simulink model "SecRwRtStFtrstTrgtPosSelc"  (R2018b)
settings: Solver=FixedStepDiscrete  StartTime=0.0  StopTime=10.0  FixedStep=0.01  RelTol=1e-3
undefined symbols (not defined in the file or in its folder): KeSMSw4SAcsMd24SecRwRtStFtrstUpwdDnwdPos_Val, KeSMSw4SAcsMd24SecRwRtStFtrstUpwdDnwdPosMax_Val, KeSMSw4SAcsMd24SecRwRtStFtrstUpwdDnwdPosMin_Val, KeSMSw4SAcsMd26SecRwRtStFtrstUpwdDnwdPos_Val, KeSMSw4SAcsMd26SecRwRtStFtrstUpwdDnwdPosMax_Val, KeSMSw4SAcsMd26SecRwRtStFtrstUpwdDnwdPosMin_Val, KeSMSw4SLegrstCloseMdSecRwRtStFtrstUpwdDnwdPos_Val, KeSMSw4SLegrstCloseMdSecRwRtStFtrstUpwdDnwdPosMax_Val, KeSMSw4SLegrstCloseMdSecRwRtStFtrstUpwdDnwdPosMin_Val, KeSMSw4SLegrstOpenMdSecRwRtStFtrstUpwdDnwdPos_Val, KeSMSw4SLegrstOpenMdSecRwRtStFtrstUpwdDnwdPosMax_Val, KeSMSw4SLegrstOpenMdSecRwRtStFtrstUpwdDnwdPosMin_Val, KeSMSw4sLyingMDSecRwRtStFtrstUpwdDnwdPos_Val, KeSMSw4sLyingMDSecRwRtStFtrstUpwdDnwdPosMax_Val, KeSMSw4sLyingMDSecRwRtStFtrstUpwdDnwdPosMin_Val, KeSMSw4sRecoveryMDSecRwRtStFtrstUpwdDnwdPos_Val, KeSMSw4sRecoveryMDSecRwRtStFtrstUpwdDnwdPosMax_Val, KeSMSw4sRecoveryMDSecRwRtStFtrstUpwdDnwdPosMin_Val, KeSMSw4sVIPMDSecRwRtStFtrstUpwdDnwdPos_Val, KeSMSw4sVIPMDSecRwRtStFtrstUpwdDnwdPosMax_Val, KeSMSw4sVIPMDSecRwRtStFtrstUpwdDnwdPosMin_Val
libraries: TrgtPosSelcLib x8
settings Model: ModifiedHistory=2023.8.1 V2.0.0 CR401790 增加模式21-26  Creator=sn2xws  LastModifiedBy=sn2xws
settings DataIOCC: SaveFormat=StructureWithTime
settings OptimizationCC: DefaultParameterBehavior=Inlined  EnhancedBackFolding=on  PassReuseOutputArgsAs=Individual arguments  ZeroExternalMemoryAtStartup=off  ZeroInternalMemoryAtStartup=off  OptimizeBlockOrder=speed  DifferentSizesBufferReuse=on  OptimizationCustomize=off
settings DebuggingCC: ParameterTunabilityLossMsg=error
settings ModelReferenceCC: ModelReferenceNumInstancesAllowed=Single
settings SFSimCC: MATLABDynamicMemAlloc=off
settings RTWCC: SystemTargetFile=autosar.tlc  GenCodeOnly=on  TemplateMakefile=ert_default_tmf  Description=AUTOSAR  GenerateReport=on  IncludeHyperlinkInReport=on  LaunchReport=on  GenerateTraceInfo=on  GenerateTraceReport=on  GenerateTraceReportSl=on  GenerateTraceReportSf=on  GenerateTraceReportEml=on
settings CodeAppCC: ForceParamTrailComments=on  IgnoreCustomStorageClasses=off  OperatorAnnotations=on  SimulinkDataObjDesc=on  SFDataObjDesc=on  InsertBlockDesc=on
settings STFCustomTargetCC: TargetLangStandard=C99 (ISO)  MultiwordLength=256  ParMdlRefBuildCompliant=on  CompOptLevelCompliant=on  IncludeMdlTerminateFcn=off  CombineOutputUpdateFcns=on  SuppressErrorStatus=on  ERTCustomFileBanners=on  SupportNonFinite=off  SupportComplex=off  SupportContinuousTime=off  SupportNonInlinedSFcns=off  RemoveResetFunc=on  MATLABClassNameForMDSCustomization=Simulink.SoftwareTarget.ERTCustomization  AutosarCompliant=on  UseToolchainInfoCompliant=on  LookupTableObjectStructAxisOrder=2,1,3,4,...  LUTObjectStructOrderEvenSpacing=Size,Table,Breakpoints  SystemTargetFile=autosar.tlc
settings ERTTargetCC: TargetLangStandard=C99 (ISO)  ConcurrentExecutionCompliant=off  IncludeMdlTerminateFcn=off  SuppressErrorStatus=on  SupportNonFinite=off  SupportComplex=off  ModelStepFunctionPrototypeControlCompliant=off  CPPClassGenCompliant=off  AutosarCompliant=on  LookupTableObjectStructAxisOrder=2,1,3,4,...  LUTObjectStructOrderEvenSpacing=Size,Table,Breakpoints  InlinedParameterPlacement=NonHierarchical  ERTCustomFileTemplate=example_file_process.tlc  ERTFilePackagingFormat=Compact

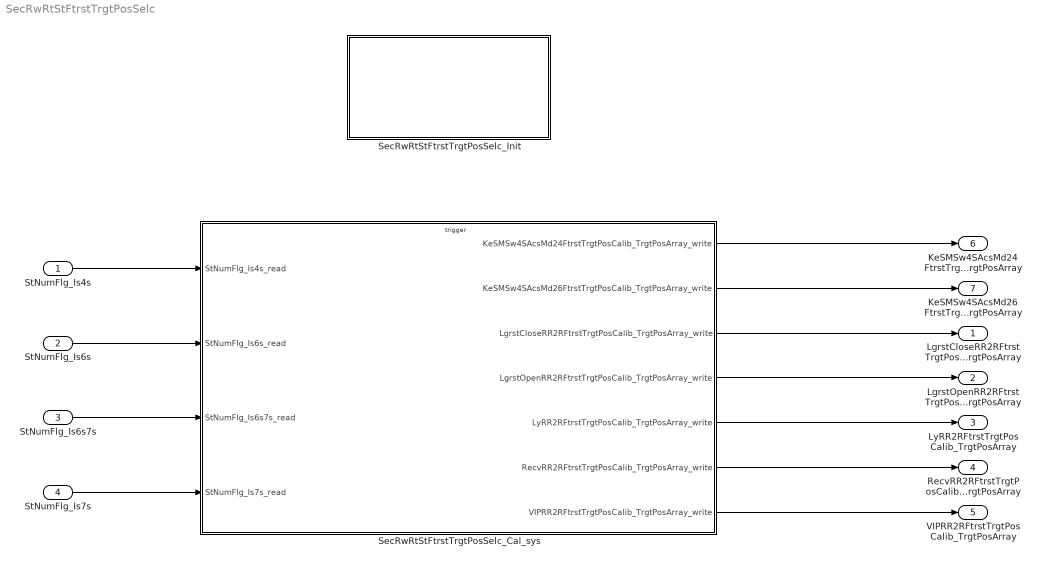
== system SecRwRtStFtrstTrgtPosSelc ==
  StNumFlg_Is4s : Inport  OutDataTypeStr=boolean  PortDimensions=1
  StNumFlg_Is6s : Inport  Port=2  OutDataTypeStr=boolean  PortDimensions=1
  StNumFlg_Is6s7s : Inport  Port=3  OutDataTypeStr=boolean  PortDimensions=1
  StNumFlg_Is7s : Inport  Port=4  OutDataTypeStr=boolean  PortDimensions=1
  SecRwRtStFtrstTrgtPosSelc_Cal_sys : Subsystem
  SecRwRtStFtrstTrgtPosSelc_Init : Subsystem
  LgrstCloseRR2RFtrstTrgtPosCalib_TrgtPosArray : Outport  Description=|  OutDataTypeStr=uint16  PortDimensions=3
      | 0:Pos
      | 1:Max
      | 2:Min
  LgrstOpenRR2RFtrstTrgtPosCalib_TrgtPosArray : Outport  Description=|  Port=2  OutDataTypeStr=uint16  PortDimensions=3
      | 0:Pos
      | 1:Max
      | 2:Min
  LyRR2RFtrstTrgtPosCalib_TrgtPosArray : Outport  Description=|  Port=3  OutDataTypeStr=uint16  PortDimensions=3
      | 0:Pos
      | 1:Max
      | 2:Min
  RecvRR2RFtrstTrgtPosCalib_TrgtPosArray : Outport  Description=|  Port=4  OutDataTypeStr=uint16  PortDimensions=3
      | 0:Pos
      | 1:Max
      | 2:Min
  VIPRR2RFtrstTrgtPosCalib_TrgtPosArray : Outport  Description=|  Port=5  OutDataTypeStr=uint16  PortDimensions=3
      | 0:Pos
      | 1:Max
      | 2:Min
  KeSMSw4SAcsMd24FtrstTrgtPosCalib_TrgtPosArray : Outport  Description=|  Port=6  OutDataTypeStr=uint16  PortDimensions=3
      | 0:Pos
      | 1:Max
      | 2:Min
  KeSMSw4SAcsMd26FtrstTrgtPosCalib_TrgtPosArray : Outport  Description=|  Port=7  OutDataTypeStr=uint16  PortDimensions=3
      | 0:Pos
      | 1:Max
      | 2:Min
  wires:
  StNumFlg_Is4s/1 -> SecRwRtStFtrstTrgtPosSelc_Cal_sys/1(StNumFlg_Is4s_read)
  StNumFlg_Is6s/1 -> SecRwRtStFtrstTrgtPosSelc_Cal_sys/2(StNumFlg_Is6s_read)
  StNumFlg_Is6s7s/1 -> SecRwRtStFtrstTrgtPosSelc_Cal_sys/3(StNumFlg_Is6s7s_read)
  StNumFlg_Is7s/1 -> SecRwRtStFtrstTrgtPosSelc_Cal_sys/4(StNumFlg_Is7s_read)
  SecRwRtStFtrstTrgtPosSelc_Cal_sys/3(LgrstCloseRR2RFtrstTrgtPosCalib_TrgtPosArray_write) -> LgrstCloseRR2RFtrstTrgtPosCalib_TrgtPosArray/1
  SecRwRtStFtrstTrgtPosSelc_Cal_sys/4(LgrstOpenRR2RFtrstTrgtPosCalib_TrgtPosArray_write) -> LgrstOpenRR2RFtrstTrgtPosCalib_TrgtPosArray/1
  SecRwRtStFtrstTrgtPosSelc_Cal_sys/5(LyRR2RFtrstTrgtPosCalib_TrgtPosArray_write) -> LyRR2RFtrstTrgtPosCalib_TrgtPosArray/1
  SecRwRtStFtrstTrgtPosSelc_Cal_sys/6(RecvRR2RFtrstTrgtPosCalib_TrgtPosArray_write) -> RecvRR2RFtrstTrgtPosCalib_TrgtPosArray/1
  SecRwRtStFtrstTrgtPosSelc_Cal_sys/7(VIPRR2RFtrstTrgtPosCalib_TrgtPosArray_write) -> VIPRR2RFtrstTrgtPosCalib_TrgtPosArray/1
  SecRwRtStFtrstTrgtPosSelc_Cal_sys/1(KeSMSw4SAcsMd24FtrstTrgtPosCalib_TrgtPosArray_write) -> KeSMSw4SAcsMd24FtrstTrgtPosCalib_TrgtPosArray/1
  SecRwRtStFtrstTrgtPosSelc_Cal_sys/2(KeSMSw4SAcsMd26FtrstTrgtPosCalib_TrgtPosArray_write) -> KeSMSw4SAcsMd26FtrstTrgtPosCalib_TrgtPosArray/1

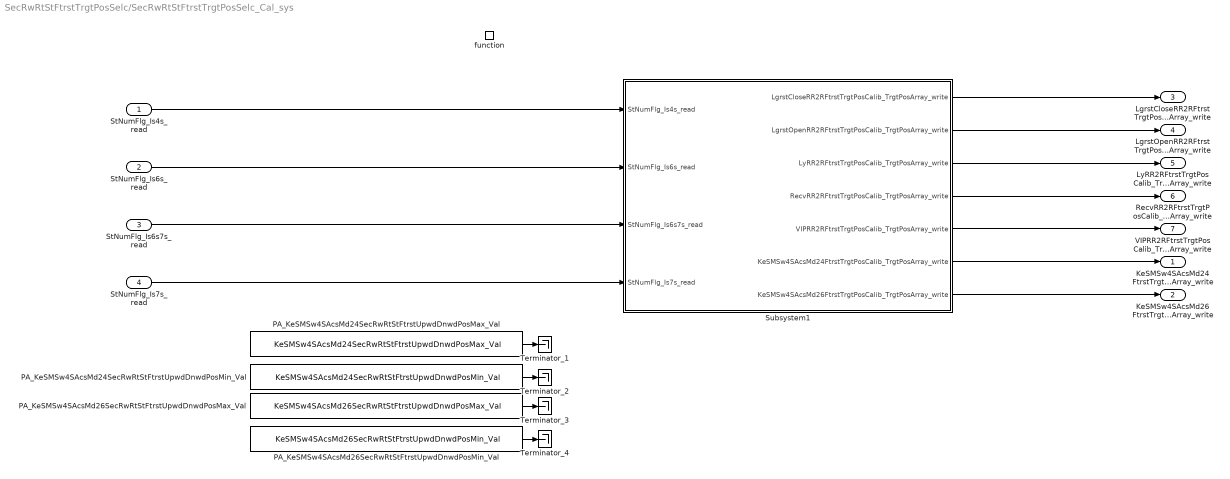
== system SecRwRtStFtrstTrgtPosSelc/SecRwRtStFtrstTrgtPosSelc_Cal_sys ==
  StNumFlg_Is4s_read : Inport
  StNumFlg_Is6s_read : Inport  Port=2
  StNumFlg_Is6s7s_read : Inport  Port=3
  StNumFlg_Is7s_read : Inport  Port=4
  function : TriggerPort  TriggerType=function-call  IsSimulinkFunction=on  FunctionName=SecRwRtStFtrstTrgtPosSelc_Cal  VariantControl=(inherit)
  PA_KeSMSw4SAcsMd24SecRwRtStFtrstUpwdDnwdPosMax_Val : Constant  Value=KeSMSw4SAcsMd24SecRwRtStFtrstUpwdDnwdPosMax_Val
  PA_KeSMSw4SAcsMd24SecRwRtStFtrstUpwdDnwdPosMin_Val : Constant  Value=KeSMSw4SAcsMd24SecRwRtStFtrstUpwdDnwdPosMin_Val
  PA_KeSMSw4SAcsMd26SecRwRtStFtrstUpwdDnwdPosMax_Val : Constant  Value=KeSMSw4SAcsMd26SecRwRtStFtrstUpwdDnwdPosMax_Val
  PA_KeSMSw4SAcsMd26SecRwRtStFtrstUpwdDnwdPosMin_Val : Constant  Value=KeSMSw4SAcsMd26SecRwRtStFtrstUpwdDnwdPosMin_Val
  Subsystem1 : Subsystem
  Terminator_{1..4} (4 alike) : Terminator
  KeSMSw4SAcsMd24FtrstTrgtPosCalib_TrgtPosArray_write : Outport
      settings: EnsureOutportIsVirtual=on
  KeSMSw4SAcsMd26FtrstTrgtPosCalib_TrgtPosArray_write : Outport  Port=2
      settings: EnsureOutportIsVirtual=on
  LgrstCloseRR2RFtrstTrgtPosCalib_TrgtPosArray_write : Outport  Port=3
      settings: EnsureOutportIsVirtual=on
  LgrstOpenRR2RFtrstTrgtPosCalib_TrgtPosArray_write : Outport  Port=4
      settings: EnsureOutportIsVirtual=on
  LyRR2RFtrstTrgtPosCalib_TrgtPosArray_write : Outport  Port=5
      settings: EnsureOutportIsVirtual=on
  RecvRR2RFtrstTrgtPosCalib_TrgtPosArray_write : Outport  Port=6
      settings: EnsureOutportIsVirtual=on
  VIPRR2RFtrstTrgtPosCalib_TrgtPosArray_write : Outport  Port=7
      settings: EnsureOutportIsVirtual=on
  wires:
  Subsystem1/1(LgrstCloseRR2RFtrstTrgtPosCalib_TrgtPosArray_write) -> LgrstCloseRR2RFtrstTrgtPosCalib_TrgtPosArray_write/1
  Subsystem1/2(LgrstOpenRR2RFtrstTrgtPosCalib_TrgtPosArray_write) -> LgrstOpenRR2RFtrstTrgtPosCalib_TrgtPosArray_write/1
  Subsystem1/3(LyRR2RFtrstTrgtPosCalib_TrgtPosArray_write) -> LyRR2RFtrstTrgtPosCalib_TrgtPosArray_write/1
  Subsystem1/4(RecvRR2RFtrstTrgtPosCalib_TrgtPosArray_write) -> RecvRR2RFtrstTrgtPosCalib_TrgtPosArray_write/1
  Subsystem1/5(VIPRR2RFtrstTrgtPosCalib_TrgtPosArray_write) -> VIPRR2RFtrstTrgtPosCalib_TrgtPosArray_write/1
  Subsystem1/6(KeSMSw4SAcsMd24FtrstTrgtPosCalib_TrgtPosArray_write) -> KeSMSw4SAcsMd24FtrstTrgtPosCalib_TrgtPosArray_write/1
  Subsystem1/7(KeSMSw4SAcsMd26FtrstTrgtPosCalib_TrgtPosArray_write) -> KeSMSw4SAcsMd26FtrstTrgtPosCalib_TrgtPosArray_write/1
  StNumFlg_Is4s_read/1 -> Subsystem1/1(StNumFlg_Is4s_read)
  StNumFlg_Is6s_read/1 -> Subsystem1/2(StNumFlg_Is6s_read)
  StNumFlg_Is6s7s_read/1 -> Subsystem1/3(StNumFlg_Is6s7s_read)
  StNumFlg_Is7s_read/1 -> Subsystem1/4(StNumFlg_Is7s_read)
  PA_KeSMSw4SAcsMd24SecRwRtStFtrstUpwdDnwdPosMax_Val/1 -> Terminator_1/1
  PA_KeSMSw4SAcsMd24SecRwRtStFtrstUpwdDnwdPosMin_Val/1 -> Terminator_2/1
  PA_KeSMSw4SAcsMd26SecRwRtStFtrstUpwdDnwdPosMax_Val/1 -> Terminator_3/1
  PA_KeSMSw4SAcsMd26SecRwRtStFtrstUpwdDnwdPosMin_Val/1 -> Terminator_4/1

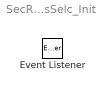
== system SecRwRtStFtrstTrgtPosSelc/SecRwRtStFtrstTrgtPosSelc_Init ==
  Event Listener : EventListener  EventName=reset

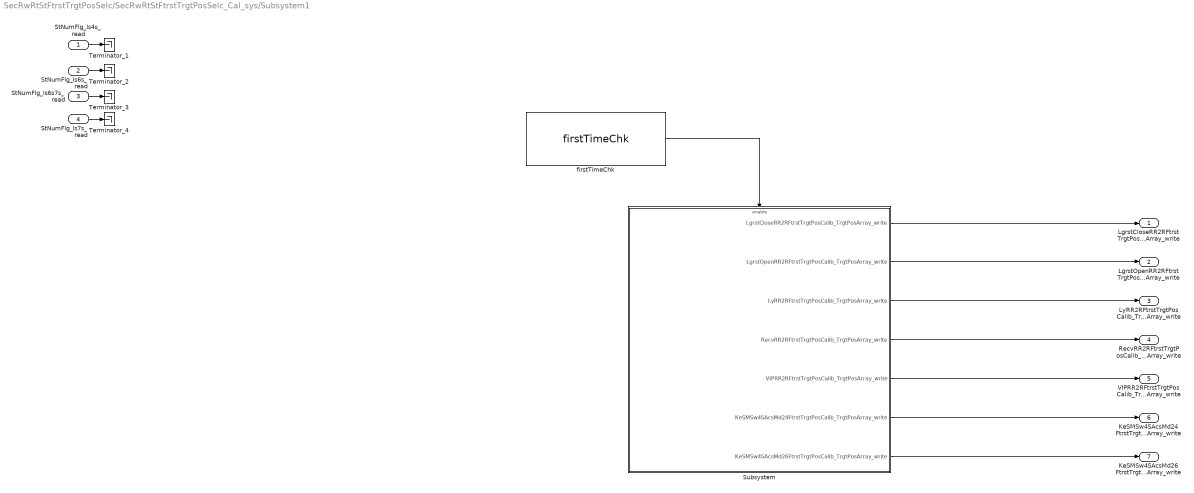
== system SecRwRtStFtrstTrgtPosSelc/SecRwRtStFtrstTrgtPosSelc_Cal_sys/Subsystem1 ==
  StNumFlg_Is4s_read : Inport
  StNumFlg_Is6s_read : Inport  Port=2
  StNumFlg_Is6s7s_read : Inport  Port=3
  StNumFlg_Is7s_read : Inport  Port=4
  Subsystem : Subsystem
  Terminator_{1..4} (4 alike) : Terminator
  firstTimeChk : TrgtPosSelcLib/firstTimeChk  SystemSampleTime=-1
  LgrstCloseRR2RFtrstTrgtPosCalib_TrgtPosArray_write : Outport
      settings: EnsureOutportIsVirtual=on
  LgrstOpenRR2RFtrstTrgtPosCalib_TrgtPosArray_write : Outport  Port=2
      settings: EnsureOutportIsVirtual=on
  LyRR2RFtrstTrgtPosCalib_TrgtPosArray_write : Outport  Port=3
      settings: EnsureOutportIsVirtual=on
  RecvRR2RFtrstTrgtPosCalib_TrgtPosArray_write : Outport  Port=4
      settings: EnsureOutportIsVirtual=on
  VIPRR2RFtrstTrgtPosCalib_TrgtPosArray_write : Outport  Port=5
      settings: EnsureOutportIsVirtual=on
  KeSMSw4SAcsMd24FtrstTrgtPosCalib_TrgtPosArray_write : Outport  Port=6
      settings: EnsureOutportIsVirtual=on
  KeSMSw4SAcsMd26FtrstTrgtPosCalib_TrgtPosArray_write : Outport  Port=7
      settings: EnsureOutportIsVirtual=on
  wires:
  StNumFlg_Is6s_read/1 -> Terminator_2/1
  Subsystem/2(LgrstOpenRR2RFtrstTrgtPosCalib_TrgtPosArray_write) -> LgrstOpenRR2RFtrstTrgtPosCalib_TrgtPosArray_write/1
  StNumFlg_Is7s_read/1 -> Terminator_4/1
  Subsystem/4(RecvRR2RFtrstTrgtPosCalib_TrgtPosArray_write) -> RecvRR2RFtrstTrgtPosCalib_TrgtPosArray_write/1
  Subsystem/1(LgrstCloseRR2RFtrstTrgtPosCalib_TrgtPosArray_write) -> LgrstCloseRR2RFtrstTrgtPosCalib_TrgtPosArray_write/1
  StNumFlg_Is6s7s_read/1 -> Terminator_3/1
  Subsystem/3(LyRR2RFtrstTrgtPosCalib_TrgtPosArray_write) -> LyRR2RFtrstTrgtPosCalib_TrgtPosArray_write/1
  StNumFlg_Is4s_read/1 -> Terminator_1/1
  firstTimeChk/1 -> Subsystem/Enable
  Subsystem/5(VIPRR2RFtrstTrgtPosCalib_TrgtPosArray_write) -> VIPRR2RFtrstTrgtPosCalib_TrgtPosArray_write/1
  Subsystem/6(KeSMSw4SAcsMd24FtrstTrgtPosCalib_TrgtPosArray_write) -> KeSMSw4SAcsMd24FtrstTrgtPosCalib_TrgtPosArray_write/1
  Subsystem/7(KeSMSw4SAcsMd26FtrstTrgtPosCalib_TrgtPosArray_write) -> KeSMSw4SAcsMd26FtrstTrgtPosCalib_TrgtPosArray_write/1

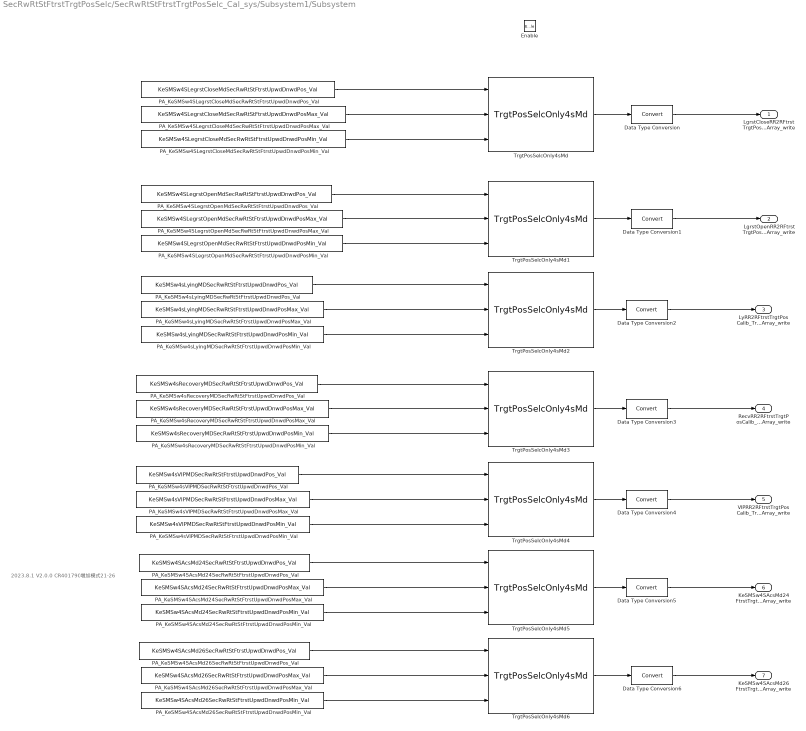
== system SecRwRtStFtrstTrgtPosSelc/SecRwRtStFtrstTrgtPosSelc_Cal_sys/Subsystem1/Subsystem ==
  note: 2023.8.1 V2.0.0 CR401790 增加模式21-26
  Enable : EnablePort
  Data Type Conversion{,1..6} (7 alike) : DataTypeConversion
  PA_KeSMSw4SAcsMd24SecRwRtStFtrstUpwdDnwdPosMax_Val : Constant  Value=KeSMSw4SAcsMd24SecRwRtStFtrstUpwdDnwdPosMax_Val
  PA_KeSMSw4SAcsMd24SecRwRtStFtrstUpwdDnwdPosMin_Val : Constant  Value=KeSMSw4SAcsMd24SecRwRtStFtrstUpwdDnwdPosMin_Val
  PA_KeSMSw4SAcsMd24SecRwRtStFtrstUpwdDnwdPos_Val : Constant  Value=KeSMSw4SAcsMd24SecRwRtStFtrstUpwdDnwdPos_Val
  PA_KeSMSw4SAcsMd26SecRwRtStFtrstUpwdDnwdPosMax_Val : Constant  Value=KeSMSw4SAcsMd26SecRwRtStFtrstUpwdDnwdPosMax_Val
  PA_KeSMSw4SAcsMd26SecRwRtStFtrstUpwdDnwdPosMin_Val : Constant  Value=KeSMSw4SAcsMd26SecRwRtStFtrstUpwdDnwdPosMin_Val
  PA_KeSMSw4SAcsMd26SecRwRtStFtrstUpwdDnwdPos_Val : Constant  Value=KeSMSw4SAcsMd26SecRwRtStFtrstUpwdDnwdPos_Val
  PA_KeSMSw4SLegrstCloseMdSecRwRtStFtrstUpwdDnwdPosMax_Val : Constant  Value=KeSMSw4SLegrstCloseMdSecRwRtStFtrstUpwdDnwdPosMax_Val
  PA_KeSMSw4SLegrstCloseMdSecRwRtStFtrstUpwdDnwdPosMin_Val : Constant  Value=KeSMSw4SLegrstCloseMdSecRwRtStFtrstUpwdDnwdPosMin_Val
  PA_KeSMSw4SLegrstCloseMdSecRwRtStFtrstUpwdDnwdPos_Val : Constant  Value=KeSMSw4SLegrstCloseMdSecRwRtStFtrstUpwdDnwdPos_Val
  PA_KeSMSw4SLegrstOpenMdSecRwRtStFtrstUpwdDnwdPosMax_Val : Constant  Value=KeSMSw4SLegrstOpenMdSecRwRtStFtrstUpwdDnwdPosMax_Val
  PA_KeSMSw4SLegrstOpenMdSecRwRtStFtrstUpwdDnwdPosMin_Val : Constant  Value=KeSMSw4SLegrstOpenMdSecRwRtStFtrstUpwdDnwdPosMin_Val
  PA_KeSMSw4SLegrstOpenMdSecRwRtStFtrstUpwdDnwdPos_Val : Constant  Value=KeSMSw4SLegrstOpenMdSecRwRtStFtrstUpwdDnwdPos_Val
  PA_KeSMSw4sLyingMDSecRwRtStFtrstUpwdDnwdPosMax_Val : Constant  Value=KeSMSw4sLyingMDSecRwRtStFtrstUpwdDnwdPosMax_Val
  PA_KeSMSw4sLyingMDSecRwRtStFtrstUpwdDnwdPosMin_Val : Constant  Value=KeSMSw4sLyingMDSecRwRtStFtrstUpwdDnwdPosMin_Val
  PA_KeSMSw4sLyingMDSecRwRtStFtrstUpwdDnwdPos_Val : Constant  Value=KeSMSw4sLyingMDSecRwRtStFtrstUpwdDnwdPos_Val
  PA_KeSMSw4sRecoveryMDSecRwRtStFtrstUpwdDnwdPosMax_Val : Constant  Value=KeSMSw4sRecoveryMDSecRwRtStFtrstUpwdDnwdPosMax_Val
  PA_KeSMSw4sRecoveryMDSecRwRtStFtrstUpwdDnwdPosMin_Val : Constant  Value=KeSMSw4sRecoveryMDSecRwRtStFtrstUpwdDnwdPosMin_Val
  PA_KeSMSw4sRecoveryMDSecRwRtStFtrstUpwdDnwdPos_Val : Constant  Value=KeSMSw4sRecoveryMDSecRwRtStFtrstUpwdDnwdPos_Val
  PA_KeSMSw4sVIPMDSecRwRtStFtrstUpwdDnwdPosMax_Val : Constant  Value=KeSMSw4sVIPMDSecRwRtStFtrstUpwdDnwdPosMax_Val
  PA_KeSMSw4sVIPMDSecRwRtStFtrstUpwdDnwdPosMin_Val : Constant  Value=KeSMSw4sVIPMDSecRwRtStFtrstUpwdDnwdPosMin_Val
  PA_KeSMSw4sVIPMDSecRwRtStFtrstUpwdDnwdPos_Val : Constant  Value=KeSMSw4sVIPMDSecRwRtStFtrstUpwdDnwdPos_Val
  TrgtPosSelcOnly4sMd{,1..6} (7 alike) : TrgtPosSelcLib/TrgtPosSelcOnly4sMd  SystemSampleTime=-1
  LgrstCloseRR2RFtrstTrgtPosCalib_TrgtPosArray_write : Outport
  LgrstOpenRR2RFtrstTrgtPosCalib_TrgtPosArray_write : Outport  Port=2
  LyRR2RFtrstTrgtPosCalib_TrgtPosArray_write : Outport  Port=3
  RecvRR2RFtrstTrgtPosCalib_TrgtPosArray_write : Outport  Port=4
  VIPRR2RFtrstTrgtPosCalib_TrgtPosArray_write : Outport  Port=5
  KeSMSw4SAcsMd24FtrstTrgtPosCalib_TrgtPosArray_write : Outport  Port=6
  KeSMSw4SAcsMd26FtrstTrgtPosCalib_TrgtPosArray_write : Outport  Port=7
  wires:
  PA_KeSMSw4sVIPMDSecRwRtStFtrstUpwdDnwdPos_Val/1 -> TrgtPosSelcOnly4sMd4/1
  PA_KeSMSw4sVIPMDSecRwRtStFtrstUpwdDnwdPosMin_Val/1 -> TrgtPosSelcOnly4sMd4/3
  PA_KeSMSw4sVIPMDSecRwRtStFtrstUpwdDnwdPosMax_Val/1 -> TrgtPosSelcOnly4sMd4/2
  TrgtPosSelcOnly4sMd3/1 -> Data Type Conversion3/1
  TrgtPosSelcOnly4sMd2/1 -> Data Type Conversion2/1
  TrgtPosSelcOnly4sMd1/1 -> Data Type Conversion1/1
  TrgtPosSelcOnly4sMd/1 -> Data Type Conversion/1
  TrgtPosSelcOnly4sMd4/1 -> Data Type Conversion4/1
  PA_KeSMSw4sRecoveryMDSecRwRtStFtrstUpwdDnwdPosMax_Val/1 -> TrgtPosSelcOnly4sMd3/2
  PA_KeSMSw4sRecoveryMDSecRwRtStFtrstUpwdDnwdPosMin_Val/1 -> TrgtPosSelcOnly4sMd3/3
  PA_KeSMSw4sRecoveryMDSecRwRtStFtrstUpwdDnwdPos_Val/1 -> TrgtPosSelcOnly4sMd3/1
  PA_KeSMSw4sLyingMDSecRwRtStFtrstUpwdDnwdPosMax_Val/1 -> TrgtPosSelcOnly4sMd2/2
  PA_KeSMSw4sLyingMDSecRwRtStFtrstUpwdDnwdPosMin_Val/1 -> TrgtPosSelcOnly4sMd2/3
  PA_KeSMSw4sLyingMDSecRwRtStFtrstUpwdDnwdPos_Val/1 -> TrgtPosSelcOnly4sMd2/1
  PA_KeSMSw4SLegrstOpenMdSecRwRtStFtrstUpwdDnwdPosMax_Val/1 -> TrgtPosSelcOnly4sMd1/2
  PA_KeSMSw4SLegrstOpenMdSecRwRtStFtrstUpwdDnwdPosMin_Val/1 -> TrgtPosSelcOnly4sMd1/3
  PA_KeSMSw4SLegrstOpenMdSecRwRtStFtrstUpwdDnwdPos_Val/1 -> TrgtPosSelcOnly4sMd1/1
  PA_KeSMSw4SLegrstCloseMdSecRwRtStFtrstUpwdDnwdPosMax_Val/1 -> TrgtPosSelcOnly4sMd/2
  PA_KeSMSw4SLegrstCloseMdSecRwRtStFtrstUpwdDnwdPosMin_Val/1 -> TrgtPosSelcOnly4sMd/3
  PA_KeSMSw4SLegrstCloseMdSecRwRtStFtrstUpwdDnwdPos_Val/1 -> TrgtPosSelcOnly4sMd/1
  Data Type Conversion/1 -> LgrstCloseRR2RFtrstTrgtPosCalib_TrgtPosArray_write/1
  Data Type Conversion1/1 -> LgrstOpenRR2RFtrstTrgtPosCalib_TrgtPosArray_write/1
  Data Type Conversion2/1 -> LyRR2RFtrstTrgtPosCalib_TrgtPosArray_write/1
  Data Type Conversion3/1 -> RecvRR2RFtrstTrgtPosCalib_TrgtPosArray_write/1
  Data Type Conversion4/1 -> VIPRR2RFtrstTrgtPosCalib_TrgtPosArray_write/1
  TrgtPosSelcOnly4sMd6/1 -> Data Type Conversion6/1
  TrgtPosSelcOnly4sMd5/1 -> Data Type Conversion5/1
  Data Type Conversion5/1 -> KeSMSw4SAcsMd24FtrstTrgtPosCalib_TrgtPosArray_write/1
  Data Type Conversion6/1 -> KeSMSw4SAcsMd26FtrstTrgtPosCalib_TrgtPosArray_write/1
  PA_KeSMSw4SAcsMd24SecRwRtStFtrstUpwdDnwdPosMin_Val/1 -> TrgtPosSelcOnly4sMd5/3
  PA_KeSMSw4SAcsMd24SecRwRtStFtrstUpwdDnwdPosMax_Val/1 -> TrgtPosSelcOnly4sMd5/2
  PA_KeSMSw4SAcsMd24SecRwRtStFtrstUpwdDnwdPos_Val/1 -> TrgtPosSelcOnly4sMd5/1
  PA_KeSMSw4SAcsMd26SecRwRtStFtrstUpwdDnwdPosMax_Val/1 -> TrgtPosSelcOnly4sMd6/2
  PA_KeSMSw4SAcsMd26SecRwRtStFtrstUpwdDnwdPosMin_Val/1 -> TrgtPosSelcOnly4sMd6/3
  PA_KeSMSw4SAcsMd26SecRwRtStFtrstUpwdDnwdPos_Val/1 -> TrgtPosSelcOnly4sMd6/1
